simulink model "svpwm_model"  (R2018a)
settings: Solver=VariableStepAuto  StartTime=0.0  StopTime=10
libraries: powerlib x25, powerlib_meascontrol x7, simulink x5
settings Model: Creator=Emre Deniz  LastModifiedBy=Emre Deniz
settings SolverCC: ZeroCrossAlgorithm=Adaptive
settings DebuggingCC: MaxConsecutiveZCsMsg=none

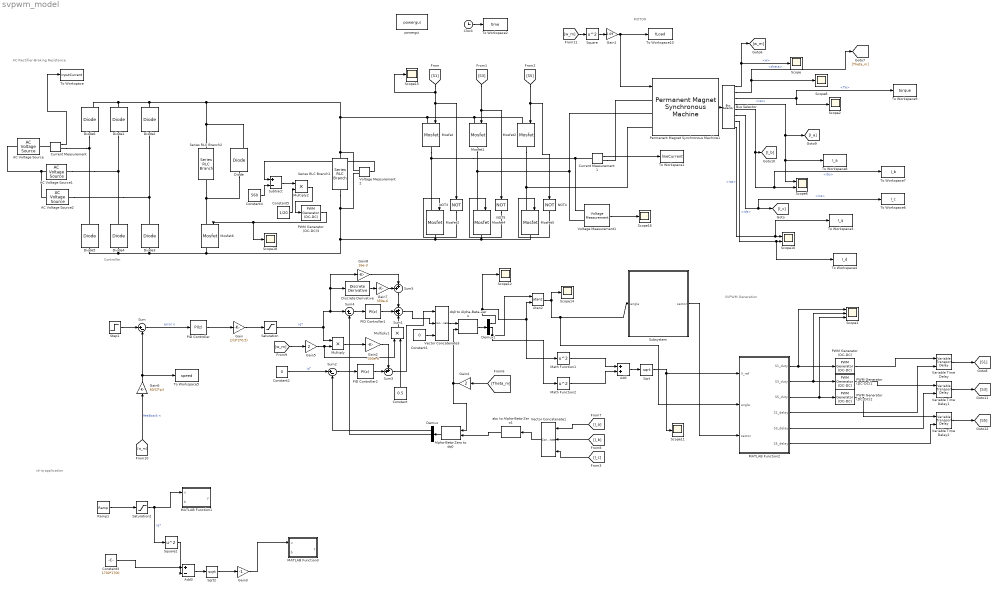
== system svpwm_model ==
  note: MOTOR
  note: Controller
  note: SVPWM Generation
  note: AC Rectifier-Braking Resistance
  note: id-iq application
  AC Voltage Source : powerlib/Electrical Sources/AC Voltage Source  Amplitude=230*sqrt(2)  Phase=0  Frequency=50  SampleTime=0  Measurements=None  BusType=swing  Pref=10e3  Qref=0  Qmin=-inf  Qmax=+inf
  AC Voltage Source1 : powerlib/Electrical Sources/AC Voltage Source  Amplitude=230*sqrt(2)  Phase=-120  Frequency=50  SampleTime=0  Measurements=None  BusType=swing  Pref=10e3  Qref=0  Qmin=-inf  Qmax=+inf
  AC Voltage Source2 : powerlib/Electrical Sources/AC Voltage Source  Amplitude=230*sqrt(2)  Phase=+120  Frequency=50  SampleTime=0  Measurements=None  BusType=swing  Pref=10e3  Qref=0  Qmin=-inf  Qmax=+inf
  Add : Sum
  Add3 : Sum  Inputs=+-
  Alpha-Beta-Zero to dq0 : powerlib_meascontrol/Transformations/Alpha-Beta-Zero to dq0  Alignment=Aligned with phase A axis
      settings: SourceProductName=Simscape Power Systems
  Atan2 : Trigonometry  Operator=atan2
  Bus Selector : BusSelector  OutputSignals=w,theta,Te,ias,ibs,ics,ids,iqs
  Clock : Clock
  Constant : Constant  Value=0.5
  Constant1 : Constant  Value=0
  Constant2 : Constant  Value=0
  Constant3 : Constant  Value=1700*1700
  Constant4 : Constant  Value=560
  Constant5 : Constant  Value=1/20
  Current Measurement : powerlib/Measurements/Current Measurement  PhasorSimulation=off  OutputType=Complex  PSBequivalent=0
  Current Measurement1 : powerlib/Measurements/Current Measurement  PhasorSimulation=off  OutputType=Complex  PSBequivalent=0
  Demux : Demux  Outputs=3
  Demux1 : Demux  Outputs=3
  Diode : powerlib/Power Electronics/Diode  Ron=0.001  Lon=0  Vf=0.8  IC=0  UseSnubber=0  Rs=500  Cs=250e-9  Measurements=on
  Diode{1..5} (5 alike) : powerlib/Power Electronics/Diode  Ron=0.001  Lon=0  Vf=0.8  IC=0  UseSnubber=0  Rs=500  Cs=250e-9  Measurements=off
  Diode6 : powerlib/Power Electronics/Diode  Ron=0.001  Lon=0  Vf=0.8  IC=0  UseSnubber=0  Rs=500  Cs=250e-9  Measurements=on
  Discrete Derivative : simulink/Quick Insert/Discrete/Discrete Derivative  gainval=1.0  ICPrevScaledInput=0.0  OutMin=[]  OutMax=[]  OutDataType=fixdt(1, 16)  OutScaling=2^-10  DoSatur=off
      settings: SourceProductName=Simulink  SourceProductBaseCode=SL
  Gain : Gain  Gain=2/(3*2*0.5)
  Gain1 : Gain  Gain=0.09
  Gain2 : Gain  Gain=-350e-6
  Gain3 : Gain  Gain=-1
  Gain4 : Gain  Gain=2
  Gain5 : Gain  Gain=2
  Gain6 : Gain  Gain=60/(2*pi)
  Gain7 : Gain  Gain=350e-6
  Gain8 : Gain  Gain=16e-3
  MATLAB Function1 : MATLAB Function  TreatAsAtomicUnit=on
  MATLAB Function2 : MATLAB Function  TreatAsAtomicUnit=on
  MATLAB Function3 : MATLAB Function  TreatAsAtomicUnit=on
  Math Function1 : Math  Operator=square  RndMeth=Zero  SaturateOnIntegerOverflow=on
  Math Function2 : Math  Operator=square  RndMeth=Zero  SaturateOnIntegerOverflow=on
  Mosfet{,1..5} (6 alike) : powerlib/Power Electronics/Mosfet  Ron=0  Lon=0  Rd=0  Vfd=0  IC=0  Rs=1e9  Cs=inf  Measurements=off
  Mosfet6 : powerlib/Power Electronics/Mosfet  Ron=0.1  Lon=0  Rd=0.01  Vfd=0  IC=0  Rs=1e5  Cs=inf  Measurements=on
  Multiply : Product
  Multiply1 : Product
  Multiply2 : Product
  NOT3 : Logic  Operator=NOT  IconShape=distinctive  AllPortsSameDT=off  OutDataTypeStr=boolean
  NOT4 : Logic  Operator=NOT  IconShape=distinctive  AllPortsSameDT=off  OutDataTypeStr=boolean
  NOT5 : Logic  Operator=NOT  IconShape=distinctive  AllPortsSameDT=off  OutDataTypeStr=boolean
  PID Controller : simulink/Continuous/PID Controller  Controller=PI  TimeDomain=Discrete-time  SampleTime=-1  IntegratorMethod=Forward Euler  FilterMethod=Forward Euler  Form=Parallel  UseFilter=on  ControllerParametersSource=internal  P=200  I=4.2  D=0  N=100  InitialConditionSource=internal  InitialConditionForIntegrator=0  InitialConditionForFilter=0  ExternalReset=none  LimitOutput=off  UpperSaturationLimit=inf  LowerSaturationLimit=-inf  LinearizeAsGain=on  AntiWindupMode=none  Kb=1  TrackingMode=off  Kt=1  PParamMin=[]  PParamMax=[]  IParamMin=[]  IParamMax=[]  DParamMin=[]  DParamMax=[]  NParamMin=[]  NParamMax=[]  KbParamMin=[]  KbParamMax=[]  KtParamMin=[]  KtParamMax=[]  POutMin=[]  POutMax=[]  IOutMin=[]  IOutMax=[]  DOutMin=[]  DOutMax=[]  NOutMin=[]  NOutMax=[]  KbOutMin=[]  KbOutMax=[]  KtOutMin=[]  KtOutMax=[]  IntegratorOutMin=[]  IntegratorOutMax=[]  FilterOutMin=[]  FilterOutMax=[]  SumOutMin=[]  SumOutMax=[]  SumI1OutMin=[]  SumI1OutMax=[]  SumI2OutMin=[]  SumI2OutMax=[]  SumI3OutMin=[]  SumI3OutMax=[]  SumDOutMin=[]  SumDOutMax=[]  SaturationOutMin=[]  SaturationOutMax=[]  IntegratorContinuousStateAttributes=''  IntegratorStateMustResolveToSignalObject=off  IntegratorRTWStateStorageClass=Auto  FilterContinuousStateAttributes=''  FilterStateMustResolveToSignalObject=off  FilterRTWStateStorageClass=Auto  DifferentiatorICPrevScaledInput=0  DifferentiatorOutMin=[]  DifferentiatorOutMax=[]  FilterDiffOutCoefMin=[]  FilterDiffOutCoefMax=[]  SumDenOutMin=[]  SumDenOutMax=[]  SumNumOutMin=[]  SumNumOutMax=[]  ReciprocalOutMin=[]  ReciprocalOutMax=[]  DivideOutMin=[]  DivideOutMax=[]  TunerSelectOption=Transfer Function Based (PID Tuner App)
  PID Controller1 : simulink/Continuous/PID Controller  Controller=PI  TimeDomain=Discrete-time  SampleTime=-1  IntegratorMethod=Forward Euler  FilterMethod=Forward Euler  Form=Ideal  UseFilter=on  ControllerParametersSource=internal  P=0.5  I=100  D=0  N=100  InitialConditionSource=internal  InitialConditionForIntegrator=0  InitialConditionForFilter=0  ExternalReset=none  LimitOutput=off  UpperSaturationLimit=inf  LowerSaturationLimit=-inf  LinearizeAsGain=on  AntiWindupMode=none  Kb=1  TrackingMode=off  Kt=1  PParamMin=[]  PParamMax=[]  IParamMin=[]  IParamMax=[]  DParamMin=[]  DParamMax=[]  NParamMin=[]  NParamMax=[]  KbParamMin=[]  KbParamMax=[]  KtParamMin=[]  KtParamMax=[]  POutMin=[]  POutMax=[]  IOutMin=[]  IOutMax=[]  DOutMin=[]  DOutMax=[]  NOutMin=[]  NOutMax=[]  KbOutMin=[]  KbOutMax=[]  KtOutMin=[]  KtOutMax=[]  IntegratorOutMin=[]  IntegratorOutMax=[]  FilterOutMin=[]  FilterOutMax=[]  SumOutMin=[]  SumOutMax=[]  SumI1OutMin=[]  SumI1OutMax=[]  SumI2OutMin=[]  SumI2OutMax=[]  SumI3OutMin=[]  SumI3OutMax=[]  SumDOutMin=[]  SumDOutMax=[]  SaturationOutMin=[]  SaturationOutMax=[]  IntegratorContinuousStateAttributes=''  IntegratorStateMustResolveToSignalObject=off  IntegratorRTWStateStorageClass=Auto  FilterContinuousStateAttributes=''  FilterStateMustResolveToSignalObject=off  FilterRTWStateStorageClass=Auto  DifferentiatorICPrevScaledInput=0  DifferentiatorOutMin=[]  DifferentiatorOutMax=[]  FilterDiffOutCoefMin=[]  FilterDiffOutCoefMax=[]  SumDenOutMin=[]  SumDenOutMax=[]  SumNumOutMin=[]  SumNumOutMax=[]  ReciprocalOutMin=[]  ReciprocalOutMax=[]  DivideOutMin=[]  DivideOutMax=[]  TunerSelectOption=Transfer Function Based (PID Tuner App)
  PID Controller2 : simulink/Continuous/PID Controller  Controller=PI  TimeDomain=Discrete-time  SampleTime=-1  IntegratorMethod=Forward Euler  FilterMethod=Forward Euler  Form=Ideal  UseFilter=on  ControllerParametersSource=internal  P=0.1  I=20  D=0  N=100  InitialConditionSource=internal  InitialConditionForIntegrator=0  InitialConditionForFilter=0  ExternalReset=none  LimitOutput=off  UpperSaturationLimit=inf  LowerSaturationLimit=-inf  LinearizeAsGain=on  AntiWindupMode=none  Kb=1  TrackingMode=off  Kt=1  PParamMin=[]  PParamMax=[]  IParamMin=[]  IParamMax=[]  DParamMin=[]  DParamMax=[]  NParamMin=[]  NParamMax=[]  KbParamMin=[]  KbParamMax=[]  KtParamMin=[]  KtParamMax=[]  POutMin=[]  POutMax=[]  IOutMin=[]  IOutMax=[]  DOutMin=[]  DOutMax=[]  NOutMin=[]  NOutMax=[]  KbOutMin=[]  KbOutMax=[]  KtOutMin=[]  KtOutMax=[]  IntegratorOutMin=[]  IntegratorOutMax=[]  FilterOutMin=[]  FilterOutMax=[]  SumOutMin=[]  SumOutMax=[]  SumI1OutMin=[]  SumI1OutMax=[]  SumI2OutMin=[]  SumI2OutMax=[]  SumI3OutMin=[]  SumI3OutMax=[]  SumDOutMin=[]  SumDOutMax=[]  SaturationOutMin=[]  SaturationOutMax=[]  IntegratorContinuousStateAttributes=''  IntegratorStateMustResolveToSignalObject=off  IntegratorRTWStateStorageClass=Auto  FilterContinuousStateAttributes=''  FilterStateMustResolveToSignalObject=off  FilterRTWStateStorageClass=Auto  DifferentiatorICPrevScaledInput=0  DifferentiatorOutMin=[]  DifferentiatorOutMax=[]  FilterDiffOutCoefMin=[]  FilterDiffOutCoefMax=[]  SumDenOutMin=[]  SumDenOutMax=[]  SumNumOutMin=[]  SumNumOutMax=[]  ReciprocalOutMin=[]  ReciprocalOutMax=[]  DivideOutMin=[]  DivideOutMax=[]  TunerSelectOption=Transfer Function Based (PID Tuner App)
  PWM Generator (DC-DC) : powerlib_meascontrol/Pulse & Signal Generators/PWM Generator (DC-DC)  Fsw=3000  Ts=1e-5
  PWM Generator (DC-DC)1 : powerlib_meascontrol/Pulse & Signal Generators/PWM Generator (DC-DC)  Fsw=3000  Ts=1e-5
  PWM Generator (DC-DC)2 : powerlib_meascontrol/Pulse & Signal Generators/PWM Generator (DC-DC)  Fsw=3000  Ts=1e-5
  PWM Generator (DC-DC)3 : powerlib_meascontrol/Pulse & Signal Generators/PWM Generator (DC-DC)  Fsw=3000  Ts=0
  Permanent Magnet Synchronous Machine1 : powerlib/Machines/Permanent Magnet Synchronous Machine  NbPhases=3  FluxDistribution=Sinusoidal  RotorType=Round  MechanicalLoad=Torque Tm  PresetModel=No  ShowDetailedParameters=on  MeasurementBus=on  Resistance=16e-3  Inductance=8.5e-3  dqInductances=[8.5e-3,8.5e-3]  La=350e-6  MachineConstant=Flux linkage established by magnets (V.s)  Flux=0.5  VoltageCst=181.3799  TorqueCst=1.5  Flat=120  Mechanical=[250 0 2 0]  PolePairs=4  InitialConditions=[141.3 ,0 , 0 , 0]  InitialConditions5ph=[0 0 0 0 0 0]  TsPowergui=0  TsBlock=-1  RefAngle=Aligned with phase A axis (original Park)
      settings: SourceProductName=Simscape Power Systems
  Ramp1 : simulink/Sources/Ramp  slope=-10  start=0  InitialOutput=1700
  Saturation : Saturate  UpperLimit=1700  LowerLimit=-1700
  Saturation2 : Saturate  UpperLimit=5000  LowerLimit=850
  Scope{,2,8,11..12,14..16,18} (9 alike) : Scope
  Scope1 : Scope  NumInputPorts=3
  Scope10 : Scope  NumInputPorts=2
  Scope6 : Scope  NumInputPorts=2
  Series RLC Branch1 : powerlib/Elements/Series RLC Branch  LConnTagsString=__new0  RConnTagsString=__new0  BranchType=C  Resistance=0.001  Inductance=1e-3  SetiL0=off  InitialCurrent=0  Capacitance=100e-3  Setx0=on  InitialVoltage=540  Measurements=None
  Series RLC Branch2 : powerlib/Elements/Series RLC Branch  LConnTagsString=__new0  RConnTagsString=__new0  BranchType=R  Resistance=1  Inductance=1e-3  SetiL0=off  InitialCurrent=0  Capacitance=1e-6  Setx0=off  InitialVoltage=0  Measurements=None
  Sqrt : Sqrt  SaturateOnIntegerOverflow=on
  Sqrt2 : Sqrt  SaturateOnIntegerOverflow=on
  Square : Math  Operator=square  SaturateOnIntegerOverflow=on
  Square2 : Math  Operator=square  SaturateOnIntegerOverflow=on
  Step1 : Step  Time=0  Before=1500  After=1500  SampleTime=0
  Subsystem : Subsystem
  Subtract : Sum  Inputs=+-
  Sum : Sum  Inputs=|+-
  Sum1 : Sum  Inputs=+++
  Sum2 : Sum  Inputs=|+-
  Sum3 : Sum  Inputs=++|
  Sum4 : Sum  Inputs=|+-
  Sum5 : Sum  Inputs=++|
  To Workspace : ToWorkspace  VariableName=inputCurrent  SaveFormat=Structure With Time  SampleTime=-1
  To Workspace1 : ToWorkspace  VariableName=lineCurrent  SaveFormat=Structure With Time  SampleTime=-1
  To Workspace10 : ToWorkspace  VariableName=tLoad  SaveFormat=Timeseries  SampleTime=-1
  To Workspace2 : ToWorkspace  VariableName=time  SampleTime=-1
  To Workspace3 : ToWorkspace  VariableName=I_q  SampleTime=-1
  To Workspace4 : ToWorkspace  VariableName=I_d  SampleTime=-1
  To Workspace5 : ToWorkspace  VariableName=speed  SampleTime=-1
  To Workspace6 : ToWorkspace  VariableName=I_c  SampleTime=-1
  To Workspace7 : ToWorkspace  VariableName=I_b  SampleTime=-1
  To Workspace8 : ToWorkspace  VariableName=I_a  SampleTime=-1
  To Workspace9 : ToWorkspace  VariableName=torque  SampleTime=-1
  Variable Time Delay : VariableTransportDelay  MaximumDelay=10
  Variable Time Delay1 : VariableTransportDelay  MaximumDelay=10
  Variable Time Delay2 : VariableTransportDelay  MaximumDelay=10
  Vector Concatenate1 : Concatenate  NumInputs=3
  Vector Concatenate3 : Concatenate  NumInputs=3
  Voltage Measurement1 : powerlib/Measurements/Voltage Measurement  PhasorSimulation=off  OutputType=Complex  PSBequivalent=0
  Voltage Measurement2 : powerlib/Measurements/Voltage Measurement  PhasorSimulation=off  OutputType=Complex  PSBequivalent=0
  abc to Alpha-Beta-Zero1 : powerlib_meascontrol/Transformations/abc to Alpha-Beta-Zero
      settings: SourceProductName=Simscape Power Systems
  dq0 to Alpha-Beta-Zero : powerlib_meascontrol/Transformations/dq0 to Alpha-Beta-Zero  Alignment=Aligned with phase A axis
      settings: SourceProductName=Simscape Power Systems  SourceProductBaseCode=PS
  powergui : powerlib/powergui  Priority=1  SimulationMode=Continuous  SampleTime=1e-5  frequency=60  Iterations=50  frequencyindice=50  Pbase=100e6  ErrMax=1e-4  UnitsV=kV  UnitsW=MW  buscounter=0  FunctionMessages=off  echomessages=off  EnableUseOfTLC=off  CurrentSourceSwitches=off  DisableSnubberDevices=off  DisableRonSwitches=off  DisableVfSwitches=off  DisplayEquations=off  SolverType=Tustin/Backward Euler (TBE)  Interpol=off  ExternalGateDelay=off  methode=off  Ts=100  x0status=blocks  SPID=on  SwTol=0  HookPort=off  RestoreLinks=warning  ResistiveCurrentMeasurement=off  Frange=[0:2:500]  Ylog=off  Xlog=on  ShowGrid=off  save=off  variable=ZData  structure=lineCurrent  ZoomFFT=off  StartTime=9  cycles=1  DisplayStyle=1  fundamental=50  FreqAxis=off  MaxFrequency=10000  frequencyindicesteady=1  RmsSteady=1  display=off
  wires:
  Step1/1 -> Sum/1
  [w_m] -> Gain6/1  "feedback n"
  Sum/1 -> PID Controller/1  "error n"
  PID Controller/1 -> Gain/1
  Gain/1 -> Saturation/1
  PID Controller1/1 -> Sum1/2
  Sum1/1 -> Vector Concatenate3/2
  Demux/1 -> Sum2/2
  Sum2/1 -> PID Controller2/1
  PID Controller2/1 -> Sum3/2
  Sum3/1 -> Vector Concatenate3/1
  Multiply/1 -> Gain2/1
  Gain2/1 -> Sum3/1
  Sum4/1 -> PID Controller1/1
  Demux/2 -> Sum4/2
  [S1] -> Scope15/1, NOT3/1, Mosfet/1
  NOT3/1 -> Mosfet3/1
  NOT5/1 -> Mosfet4/1
  NOT4/1 -> Mosfet5/1
  [S3] -> NOT5/1, Mosfet1/1
  [S5] -> NOT4/1, Mosfet2/1
  Permanent Magnet Synchronous Machine1/1 -> Bus Selector/1
  Bus Selector/1 -> [w_m], Scope/1  "<w>"
  Bus Selector/2 -> [Theta_m], Scope8/1  "<theta>"
  [Theta_m] -> Gain4/1
  Gain4/1 -> dq0 to Alpha-Beta-Zero/2, Alpha-Beta-Zero to dq0/2
  Bus Selector/4 -> To Workspace8/1, Scope6/1, [I_a]  "<ias>"
  Bus Selector/5 -> To Workspace7/1, Scope6/2, [I_b]  "<ibs>"
  [I_a] -> Vector Concatenate1/1
  [I_b] -> Vector Concatenate1/2
  [w_m] -> Gain5/1
  Gain5/1 -> Multiply1/1, Multiply/2
  Multiply1/1 -> Sum1/3
  Constant/1 -> Multiply1/2
  [w_m] -> Square/1
  Square/1 -> Gain1/1
  Bus Selector/3 -> Scope2/1, To Workspace9/1  "<Te>"
  Discrete Derivative/1 -> Gain7/1
  Gain7/1 -> Sum5/1
  Sum5/1 -> Sum1/1
  Gain8/1 -> Sum5/2
  Demux1/2 -> Atan2/1, Math Function2/1
  Demux1/1 -> Scope12/1, Atan2/2, Math Function1/1
  Atan2/1 -> MATLAB Function2/2(angle), Subsystem/1(angle), Scope14/1
  Math Function2/1 -> Add/2
  Math Function1/1 -> Add/1
  Add/1 -> Sqrt/1
  Subsystem/1("sector ") -> MATLAB Function2/3(sector)
  Voltage Measurement1/1 -> Scope16/1
  MATLAB Function2/1(S1_duty) -> Scope1/1, PWM Generator (DC-DC)/1
  MATLAB Function2/4(S1_delay) -> Variable Time Delay/2
  MATLAB Function2/5(S3_delay) -> Variable Time Delay1/2
  MATLAB Function2/6(S5_delay) -> Variable Time Delay2/2
  Variable Time Delay/1 -> [S1]
  Variable Time Delay1/1 -> [S3]
  Variable Time Delay2/1 -> [S5]
  PWM Generator (DC-DC)/1 -> Variable Time Delay/1
  PWM Generator (DC-DC)1/1 -> Variable Time Delay1/1
  PWM Generator (DC-DC)2/1 -> Variable Time Delay2/1
  MATLAB Function2/2(S3_duty) -> Scope1/2, PWM Generator (DC-DC)1/1
  MATLAB Function2/3(S5_duty) -> Scope1/3, PWM Generator (DC-DC)2/1
  Current Measurement/1 -> To Workspace/1
  Bus Selector/6 -> To Workspace6/1, [I_c]  "<ics>"
  [I_c] -> Vector Concatenate1/3
  Vector Concatenate1/1 -> abc to Alpha-Beta-Zero1/1
  abc to Alpha-Beta-Zero1/1 -> Alpha-Beta-Zero to dq0/1
  Alpha-Beta-Zero to dq0/1 -> Demux/1
  Sqrt/1 -> MATLAB Function2/1(V_ref), Scope11/1
  Constant1/1 -> Vector Concatenate3/3
  Vector Concatenate3/1 -> dq0 to Alpha-Beta-Zero/1
  dq0 to Alpha-Beta-Zero/1 -> Demux1/1
  Clock/1 -> To Workspace2/1
  Gain1/1 -> To Workspace10/1, Permanent Magnet Synchronous Machine1/1
  Bus Selector/7 -> To Workspace4/1, Scope10/2  "<ids>"
  Bus Selector/8 -> To Workspace3/1, Scope10/1  "<iqs>"
  Gain6/1 -> Sum/2, To Workspace5/1
  Saturation2/1 -> MATLAB Function1/1(u), Square2/1  "iq*"
  Constant3/1 -> Add3/1
  Ramp1/1 -> Saturation2/1
  Square2/1 -> Add3/2
  Add3/1 -> Sqrt2/1
  Sqrt2/1 -> Gain3/1
  Gain3/1 -> MATLAB Function3/1(u)
  Constant2/1 -> Sum2/1  "id\""
  Saturation/1 -> Multiply/1, Gain8/1, Discrete Derivative/1, Sum4/1  "iq*"
  PWM Generator (DC-DC)3/1 -> Scope18/1, Mosfet6/1
  Multiply2/1 -> PWM Generator (DC-DC)3/1
  Voltage Measurement2/1 -> Subtract/1
  Constant4/1 -> Subtract/2
  Constant5/1 -> Multiply2/2
  Subtract/1 -> Multiply2/1
  Current Measurement1/1 -> To Workspace1/1
  ? -> MATLAB Function1/2(b)
  connections:
  Diode6/LConn1 -- Current Measurement/RConn1 -- Diode5/RConn1
  AC Voltage Source1/RConn1 -- Diode4/RConn1 -- Diode1/LConn1
  AC Voltage Source2/RConn1 -- Diode3/RConn1 -- Diode2/LConn1
  AC Voltage Source2/LConn1 -- AC Voltage Source/LConn1 -- AC Voltage Source1/LConn1
  Mosfet/RConn1 -- Voltage Measurement1/LConn1 -- Current Measurement1/LConn1 -- Mosfet3/LConn1
  Mosfet1/RConn1 -- Voltage Measurement1/LConn2 -- Permanent Magnet Synchronous Machine1/LConn2 -- Mosfet4/LConn1
  Mosfet2/RConn1 -- Permanent Magnet Synchronous Machine1/LConn3 -- Mosfet5/LConn1
  Current Measurement/LConn1 -- AC Voltage Source/RConn1
  Current Measurement1/RConn1 -- Permanent Magnet Synchronous Machine1/LConn1
  Series RLC Branch1/LConn1 -- Mosfet2/LConn1 -- Mosfet1/LConn1 -- Mosfet/LConn1 -- Series RLC Branch2/LConn1 -- Diode/RConn1 -- Diode1/RConn1 -- Diode6/RConn1 -- Diode2/RConn1 -- Voltage Measurement2/LConn1
  Series RLC Branch1/RConn1 -- Diode5/LConn1 -- Diode4/LConn1 -- Diode3/LConn1 -- Mosfet6/RConn1 -- Mosfet3/RConn1 -- Mosfet5/RConn1 -- Mosfet4/RConn1 -- Voltage Measurement2/LConn2
  Mosfet6/LConn1 -- Series RLC Branch2/RConn1 -- Diode/LConn1

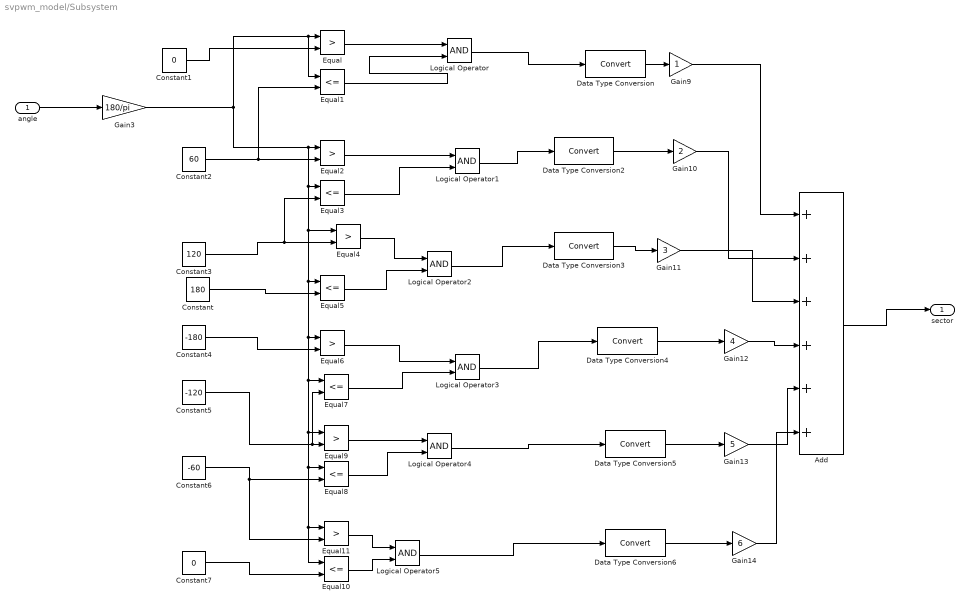
== system svpwm_model/Subsystem ==
  angle : Inport
  Add : Sum  Inputs=++++++
  Constant : Constant  Value=180
  Constant1 : Constant  Value=0
  Constant2 : Constant  Value=60
  Constant3 : Constant  Value=120
  Constant4 : Constant  Value=-180
  Constant5 : Constant  Value=-120
  Constant6 : Constant  Value=-60
  Constant7 : Constant  Value=0
  Data Type Conversion{,2..6} (6 alike) : DataTypeConversion
  Equal{,2,4,6,9,11} (6 alike) : RelationalOperator  Operator=>  OutDataTypeStr=boolean  RndMeth=Simplest
  Equal{1,3,5,7..8,10} (6 alike) : RelationalOperator  Operator=<=  OutDataTypeStr=boolean  RndMeth=Simplest
  Gain10 : Gain  Gain=2
  Gain11 : Gain  Gain=3
  Gain12 : Gain  Gain=4
  Gain13 : Gain  Gain=5
  Gain14 : Gain  Gain=6
  Gain3 : Gain  Gain=180/pi
  Gain9 : Gain
  Logical Operator{,1..5} (6 alike) : Logic  AllPortsSameDT=off  OutDataTypeStr=boolean
  "sector " : Outport
  wires:
  Gain3/1 -> Equal10/1, Equal11/1, Equal8/1, Equal9/1, Equal7/1, Equal6/1, Equal5/1, Equal4/1, Equal3/1, Equal2/1, Equal1/1, Equal/1
  Constant3/1 -> Equal3/2, Equal4/2
  Equal5/1 -> Logical Operator2/2
  Logical Operator4/1 -> Data Type Conversion5/1
  Constant6/1 -> Equal8/2, Equal11/2
  Data Type Conversion/1 -> Gain9/1
  Gain11/1 -> Add/3
  Logical Operator/1 -> Data Type Conversion/1
  Constant2/1 -> Equal1/2, Equal2/2
  Gain10/1 -> Add/2
  Equal10/1 -> Logical Operator5/2
  Logical Operator5/1 -> Data Type Conversion6/1
  Constant4/1 -> Equal6/2
  Equal4/1 -> Logical Operator2/1
  Equal11/1 -> Logical Operator5/1
  Gain14/1 -> Add/6
  Add/1 -> "sector "/1
  Logical Operator1/1 -> Data Type Conversion2/1
  Logical Operator3/1 -> Data Type Conversion4/1
  angle/1 -> Gain3/1
  Gain12/1 -> Add/4
  Data Type Conversion6/1 -> Gain14/1
  Data Type Conversion2/1 -> Gain10/1
  Equal9/1 -> Logical Operator4/1
  Constant1/1 -> Equal/2
  Equal8/1 -> Logical Operator4/2
  Constant7/1 -> Equal10/2
  Equal/1 -> Logical Operator/1
  Equal3/1 -> Logical Operator1/2
  Constant5/1 -> Equal7/2, Equal9/2
  Data Type Conversion5/1 -> Gain13/1
  Equal1/1 -> Logical Operator/2
  Gain9/1 -> Add/1
  Logical Operator2/1 -> Data Type Conversion3/1
  Equal6/1 -> Logical Operator3/1
  Equal7/1 -> Logical Operator3/2
  Gain13/1 -> Add/5
  Equal2/1 -> Logical Operator1/1
  Data Type Conversion3/1 -> Gain11/1
  Data Type Conversion4/1 -> Gain12/1
  Constant/1 -> Equal5/2

== matlab function svpwm_model/MATLAB Function1 ==
  data: u input; y output; b input
function y = fcn(u,b)
if b > 2250
    y = 848;
else
    y = u;
end

== matlab function svpwm_model/MATLAB Function3 ==
  data: u input; y output; b input
function y = fcn(u,b)
if b > 2250
    y = 0;
else
    y = u;
end

== matlab function svpwm_model/MATLAB Function2 ==
  data: V_ref input; S1_duty output; angle input; sector input; S3_duty output; S5_duty output; S1_delay output; S3_delay output; S5_delay output
function [S1_duty, S3_duty, S5_duty, S1_delay, S3_delay, S5_delay]= fcn(V_ref, angle, sector)

V_max = 540 * 1 / sqrt(3);

if(V_ref > V_max)
    V_ref = V_max-0.1;
end

T_1 = 0;
T_2 = T_1;
T_3 = T_2;
T_4 = T_3;
T_5 = T_4;
T_6 = T_5;
f = 3000;
Ts = 1/f;
zero_switch_ratio = 1 - V_ref / V_max;
T_zero = Ts* ( 1 - V_ref / V_max);
T_0 = T_zero / 2 ;
T_7 = T_0;
S1_duty = 0;
S3_duty = 0;
S5_duty = 0;
S1_delay = 0;
S3_delay = 0;
S5_delay = 0;



if sector == 1
    angle = angle;
    T_ratio = sin(angle) / sin(pi/3-angle);
    T_vector = Ts - T_zero;
    T_second = T_ratio * (T_vector/(T_ratio + 1));
    T_first = T_vector - T_second;
    T_1 = T_first;
    T_2 = T_second;
    
    S1_delay = T_0/2;
    S3_delay = T_0/2 + T_1/2;
    S5_delay = T_0/2 + T_1/2 + T_2/2;
    
    S1_duty = (Ts - T_0) / Ts;
    S3_duty = (Ts - T_1 - T_0 ) / Ts;
    S5_duty = (Ts - T_1 - T_0 - T_2) / Ts;
   
    
elseif sector == 2
    angle = angle - pi/3;
    T_ratio = sin(angle) / sin(pi/3-angle);
    T_vector = Ts - T_zero;
    T_second = T_ratio * (T_vector/(T_ratio + 1));
    T_first = T_vector - T_second;
    T_2 = T_first;
    T_3 = T_second;
    
    
    S3_delay = T_0/2;
    S1_delay = T_0/2 + T_3/2;
    S5_delay = T_0/2 + T_3/2 + T_2/2 ;
    
    
    S3_duty = (Ts - T_0) / Ts;
    S1_duty = (Ts - T_3 - T_0) / Ts;
    S5_duty = (Ts - T_2 - T_3 - T_0) / Ts;
   
elseif sector == 3
    
   
    angle = angle - 2*pi/3;
    T_ratio = sin(angle) / sin(pi/3-angle);
    T_vector = Ts - T_zero;
    T_second = T_ratio * (T_vector/(T_ratio + 1));
    T_first = T_vector - T_second;
    T_3 = T_first;
    T_4 = T_second;
    
    S3_delay = T_0/2;
    S5_delay = T_0/2 + T_3/2;
    S1_delay = T_0/2 + T_3/2 + T_4/2;
    
    S3_duty = (Ts - T_0) / Ts;
    S5_duty = (Ts - T_3 - T_0) / Ts;
    S1_duty = (Ts - T_4 - T_3 - T_0) / Ts;
    
elseif sector == 4
    angle = angle - pi;
    T_ratio = sin(angle) / sin(pi/3-angle);
    T_vector = Ts - T_zero;
    T_second = T_ratio * (T_vector/(T_ratio + 1));
    T_first = T_vector - T_second;
    T_4 = T_first;
    T_5 = T_second;
    
    S5_delay = T_0/2;
    S3_delay = T_0/2 + T_5/2;
    S1_delay = T_0/2 + T_5/2 + T_4/2;
    
    S5_duty = (Ts - T_0) / Ts;
    S3_duty = (Ts - T_5 - T_0) / Ts;
    S1_duty = (Ts - T_4 - T_5 - T_0) / Ts;
    
    
elseif sector == 5
    angle = angle - 4*pi/3;
    T_ratio = sin(angle) / sin(pi/3-angle);
    T_vector = Ts - T_zero;
    T_second = T_ratio * (T_vector/(T_ratio + 1));
    T_first = T_vector - T_second;
    T_5 = T_first;
    T_6 = T_second;
    
    S5_delay = T_0/2;
    S1_delay = T_0/2 + T_5/2;
    S3_delay = T_0/2 + T_5/2 + T_6/2;
    
    S5_duty = (Ts - T_0) / Ts;
    S1_duty = (Ts - T_5 - T_0) / Ts;
    S3_duty = (Ts - T_6 - T_5 - T_0) / Ts;
else
    angle = angle - 5*pi/3;
    T_ratio = sin(angle) / sin(pi/3-angle);
    T_vector = Ts - T_zero;
    T_second = T_ratio * (T_vector/(T_ratio + 1));
    T_first = T_vector - T_second;
    T_6 = T_first;
    T_1 = T_second;
    
    S1_delay = T_0/2;
    S5_delay = T_0/2 + T_1/2;
    S3_delay = T_0/2 + T_1/2 + T_6/2;
    
    S1_duty = (Ts - T_0) / Ts;
    S5_duty = (Ts - T_1 - T_0) / Ts;
    S3_duty = (Ts - T_6 - T_1 - T_0) / Ts;
    
end
